simulink model "PubIfDecisionTOS_MDL"  (R2020b)
settings: configuration reference "DspaceConfig" (kept outside this file)
PostLoadFcn:
  | if any(exist('dsrtsu_mdlpostloadfcn', 'file') ~= 0), dsrtsu_mdlpostloadfcn('Execute', bdroot); end
InitFcn:
  | , if any(exist('dsmpb_private', 'file') ~= 0), dsmpb_private('dsmpb_mdlclblib', 'Init', bdroot); end,
undefined symbols (not defined in the file or in its folder): C_TOS_ACCEgoRAxletoFbumplength_m, C_TOS_ACCTargetFront_Flag, C_TOS_AEBJAPedObjDxThre_Val, C_TOS_AEBJAPedObjDyThre_Val, C_TOS_AEBJATargetSize_Val, C_TOS_AEBJAVehObjDxThre_Val, C_TOS_AEBJAVehObjDyThre_Val, C_TOS_AEBJuncPedTargetSize_Val, C_TOS_AEBLatObjDxThre_Val, C_TOS_AEBLatPedDyThre_Val, C_TOS_AEBLatTargetSize_Val, C_TOS_AEBLongTargetInEgoFront_Flag, C_TOS_axAbsGround_Parameter, C_TOS_CameraConfirmedFlag, C_TOS_CNsubjWidth, C_TOS_CurrentLaneCoreMinWidth_Val, C_TOS_CutInProb_Val_Zero, C_TOS_CutOutProb_Val_Zero, C_TOS_D2R_Val, C_TOS_DefaultValueObjectToCenterLine_dy, C_TOS_EgoCarWidth_Val, C_TOS_EgoDxRefPoint_m, C_TOS_EgoRAxletoFbumplength_m, C_TOS_HalfWidthVehicle_Con, C_TOS_HWA_CurrentLaneFlag, C_TOS_HWA_LeftLaneFlag, C_TOS_HWA_MovingDir_Vaild, C_TOS_HWA_MovState_Vaild, C_TOS_HWA_RightLaneFlag, C_TOS_LaneLineCourseErrorFront, C_TOS_LaneLineCourseErrorRear, C_TOS_MotorbikeDefaultWidth_m, C_TOS_NumberOfEffectiveTargets, C_TOS_Obj_Age_Val, C_TOS_Objdx_Constraint_Val, C_TOS_ObjectDefaultWidth_m, C_TOS_ObjInCurrentLane_Val, C_TOS_ObjInCurrentLaneValid, C_TOS_ObjInLeftLaneValid, C_TOS_ObjInRightLaneValid, C_TOS_ObjNotInCurrentLane_Val, C_TOS_ObjNotREElementType, C_TOS_ObjPredictDis_dy_ConstantVal_Zeros, C_TOS_ObjToCenterLine_ConstantVal_Zeros, C_TOS_OFMObjIDInvilad_Val, C_TOS_PIL_LatDisCons_Val_zero, C_TOS_PIL_ObjectCutInFlag_b, C_TOS_PIL_ObjectCutOutFlag_b, C_TOS_PIL_ObjLaneProb_al_Val, C_TOS_PP_ObjFusType_FC_Confirm_b, C_TOS_PP_ObjFusType_FC_FR_Confirm_b, C_TOS_PP_ObjFusType_FR_Confirm_b, C_TOS_RE_80BoolDefault_Val, C_TOS_RE_80Single181Default_Val, C_TOS_RE_80Single255Default_Val, C_TOS_RE_80Uint8Default_Val, C_TOS_RE_D2R, C_TOS_RE_D_180_Val, C_TOS_RE_InvalidObjectID_Val, C_TOS_RE_InvalidTargetChainDir_Val ... (+142)
libraries: simulink x1650, TOS_LIB x361, canfdmsglib x14
(part 67 of 69)

== stateflow chart PubIfDecisionTOS_MDL/TOS_20201112/TOS_2012080320/PP1128/AAT-AdditionalAttributes/RoadEdge/RE_2020_12_07/RoadEdge_V2/TargetChain/ObjectIsTargetChainElement/EgoLeft_TargetChainElementJudge ==
  state TargetChainElementJudge [function]
    (default) -> (junction 511) : {
        | OFM_Target_Index_i = RE_StationaryObjectsSortIndex[i] - uint8(1);
        | OFM_Target_Index_i_1  = RE_StationaryObjectsSortIndex[i- uint8(1)] - uint8(1);
        |  }
        | %OFM目标的 Index,从0开始
    (junction 511) -> (junction 327)
    (junction 327) -> (junction 333) [order 1] : [(i == uint8(1)&&RE_TargetChainStartDirection[i] == uint8(1))||...
        | RE_TargetChainDirection[i] == uint8(1)||...
        | RE_TargetChainDirection[i] == uint8(3)||...
        | RE_TargetChainDirection[i] == uint8(5)]
    (junction 327) -> (junction 357) [order 2]
    (junction 333) -> (junction 337)
    (junction 337) -> (junction 332) [order 1] : [abs(Object_Dx[OFM_Target_Index_i] - Object_Dx[OFM_Target_Index_i_1]) < P_TOS_RE_SameDirTargetChainDxThre_Val&&...
        | abs(Object_Dy[OFM_Target_Index_i] - Object_Dy[OFM_Target_Index_i_1]) <P_TOS_RE_SameDirTargetChainDyThre_Val]
    (junction 357) -> (junction 352) [order 1] : [(i == uint8(1)&&(RE_TargetChainStartDirection[i] == uint8(2)||...
        | RE_TargetChainStartDirection[i] == uint8(3)))||...
        | RE_TargetChainDirection[i] == uint8(2)||...
        | RE_TargetChainDirection[i] == uint8(4)||...
        | RE_TargetChainDirection[i] == uint8(6)]
    (junction 332) -> (junction 353) : {
        | RE_TargetChainElementFlag[i] = true;
        | }
    (junction 352) -> (junction 349)
    (junction 337) -> (junction 331) [order 2] : {
        | RE_TargetChainElementFlag[i] = false;
        | }
    (junction 357) -> (junction 336) [order 2] : {
        | RE_TargetChainElementFlag[i] = false;
        | }
    (junction 349) -> (junction 356) [order 1] : [abs(Object_Dx[OFM_Target_Index_i] - Object_Dx[OFM_Target_Index_i_1] )< P_TOS_RE_DiffDirTargetChainDxThre_Val&&...
        | abs(Object_Dy[OFM_Target_Index_i] - Object_Dy[OFM_Target_Index_i_1] )<P_TOS_RE_DiffDirTargetChainDyThre_Val]
    (junction 349) -> (junction 355) [order 2] : {
        | RE_TargetChainElementFlag[i] = false;
        | }
    (junction 356) -> (junction 329) : {
        | RE_TargetChainElementFlag[i] = true;
        | }
    (junction 355) -> (junction 336)
    (junction 329) -> (junction 355)
    (junction 331) -> (junction 329)
    (junction 353) -> (junction 331)
    (junction 336) -> (junction 460)
  state TargetChainNumCal [function]
    note: 计算连续满足条件的元素个数
    note: 3个目标组成一条链目标连；
        | 计算得到目标链的起始目标在Dx排序中的Index+1；
    (default) -> (junction 372)
    (junction 372) -> (junction 378) [order 1] : [RE_TargetChainElementFlag[i] == true]
    (junction 372) -> (junction 379) [order 2] : {
        | ElementCounter[i] = uint8(0);
        | }
    (junction 378) -> (junction 396) : {
        | ElementCounter[i] = ElementCounter[i-uint8(1)] + uint8(1);
        | }
    (junction 396) -> (junction 379)
    (junction 379) -> (junction 369)
    (junction 369) -> (junction 382) [order 1] : [ElementCounter[i] == uint8(2)]
        | %连续2个目标符合条件时，从起始目标到当前目标一共是3个目标；
    (junction 369) -> (junction 375) [order 2]
    (junction 382) -> (junction 376) : {
        | TargetChainStartIndex[i - uint8(2)] = i - uint8(1);
        | TargetChainStartIndex[i - uint8(1)] = i - uint8(1);
        | TargetChainStartIndex[i] = i - uint8(1);
        | %ElementCounter[i - uint8(2)] == uint8(1);
        | %ElementCounter[i - uint8(1)] == uint8(2);
        | %目标链开始元素从1开始计数
        | }
    (junction 375) -> (junction 373) [order 1] : [ElementCounter[i] > uint8(2)]
    (junction 375) -> (junction 377) [order 2] : {
        | TargetChainStartIndex[i] = uint8(0);
        | %ElementCounter[i] = uint8(0);
        | }
    (junction 373) -> (junction 387) : {
        | TargetChainStartIndex[i] = TargetChainStartIndex[i - uint8(1)];
        | }
    (junction 387) -> (junction 377)
    (junction 376) -> (junction 387)
    (junction 377) -> (junction 495)
  (default) -> (junction 2) : {
      | i = uint8(1);
      | RE_TargetChainElementFlag = C_TOS_RE_80BoolDefault_Val;
      | TargetChainStartIndex = C_TOS_RE_80Uint8Default_Val;
      | ElementCounter = C_TOS_RE_80Uint8Default_Val;
      | }
      | %从第2个目标开始
  (junction 2) -> (junction 3) [order 1] : [RE_StationaryObjectsSortIndex[i] ~= C_TOS_StillObjSortInvalidIndex_Val&&...
      | i <= uint8(79)]
  (junction 360) -> (junction 2) : {
      | i = i+uint8(1);
      | }
  (junction 2) -> (junction 314) [order 2]
  (junction 3) -> (junction 358) : {
      | TargetChainElementJudge();
      | }
  (junction 358) -> (junction 360) : {
      | TargetChainNumCal();
      | }
  (junction 314) -> (junction 8)
  data: C_TOS_RE_InvalidTargetChainDir_Val parameter; C_TOS_StillObjSortInvalidIndex_Val parameter; Object_Dx input; Object_Dy input; P_TOS_RE_DiffDirTargetChainDxThre_Val parameter; P_TOS_RE_DiffDirTargetChainDyThre_Val parameter; P_TOS_RE_SameDirTargetChainDxThre_Val parameter; P_TOS_RE_SameDirTargetChainDyThre_Val parameter; RE_StationaryObjectsSortIndex input; RE_TargetChainDirection input; RE_TargetChainStartDirection input; i local uint8 =; RE_TargetChainElementFlag output boolean size=80; TargetChainStartIndex output uint8 size=80; OFM_Target_Index_i local uint8 size=1; k local uint8; TargetChainNum local uint8; OFM_Target_Index_i_1 local uint8 size=1; C_TOS_RE_80BoolDefault_Val parameter; C_TOS_RE_80Uint8Default_Val parameter; ElementCounter output uint8 size=80 =

== stateflow chart PubIfDecisionTOS_MDL/TOS_20201112/TOS_2012080320/PP1128/AAT-AdditionalAttributes/RoadEdge/RE_2020_12_07/RoadEdge_V2/TargetChain/ObjectIsTargetChainElement/EgoLeft_TargetChainInfor ==
  state TargetChainNumCal [function]
    note: 给目标链编号
    (default) -> (junction 473) : %目标链条数从1开始
    (junction 473) -> (junction 482) [order 1] : [i == uint8(0)]
    (junction 473) -> (junction 374) [order 2]
    (junction 482) -> (junction 481)
    (junction 374) -> (junction 383) [order 1] : [(TargetChainStartIndex[i-uint8(1)] == uint8(0)&&...
        | TargetChainStartIndex[i] != uint8(0))||...
        | (TargetChainStartIndex[i-uint8(1)] != uint8(0)&&...
        | TargetChainStartIndex[i] != uint8(0)&&...
        | TargetChainStartIndex[i] != TargetChainStartIndex[i-uint8(1)])]
        | %目标链开始元素
    (junction 481) -> (junction 475) [order 1] : [TargetChainStartIndex[i] != uint8(0)]
        | %Dx最近的目标是目标链开始元素
    (junction 374) -> (junction 365) [order 2]
    (junction 383) -> (junction 391) : {
        | TargetChainIndex[i] = TargetChainNum;
        |  TargetChainNum = TargetChainNum + uint8(1);
        | }
    (junction 481) -> (junction 486) [order 2] : {
        | TargetChainIndex[i] = uint8(0);
        | }
    (junction 475) -> (junction 477) : {
        | TargetChainIndex[i] = TargetChainNum;
        |  TargetChainNum = TargetChainNum + uint8(1);
        | }
    (junction 365) -> (junction 414) [order 1] : [TargetChainStartIndex[i] != uint8(0)&&...
        | TargetChainStartIndex[i] == TargetChainStartIndex[i-uint8(1)]]
        | %目标链剩余元素
    (junction 365) -> (junction 381) [order 2] : {
        | TargetChainIndex[i] = uint8(0);
        | }
    (junction 414) -> (junction 368) : {
        | TargetChainIndex[i] = TargetChainIndex[i-uint8(1)];
        | }
    (junction 368) -> (junction 381)
    (junction 391) -> (junction 368)
    (junction 486) -> (junction 391)
    (junction 477) -> (junction 486)
    (junction 381) -> (junction 501)
  state TargetChainElementNumCal [function]
    (default) -> (junction 517)
    (junction 517) -> (junction 516) [order 1] : [i > uint8(0)]
    (junction 517) -> (junction 520) [order 2] : {
        | TargetChainElementNum[i] = uint8(0);
        | }
    (junction 516) -> (junction 437)
    (junction 437) -> (junction 448) [order 1] : [(TargetChainStartIndex[i-uint8(1)] != uint8(0)&&...
        | TargetChainStartIndex[i] == uint8(0))||...
        | (TargetChainStartIndex[i-uint8(1)] != uint8(0)&&...
        | TargetChainStartIndex[i] != TargetChainStartIndex[i-uint8(1)])]
        | %[i-uint8(1)]为目标链结束元素
    (junction 437) -> (junction 442) [order 2] : {
        | TargetChainElementNum[i-uint8(1)] = uint8(0);
        | }
    (junction 448) -> (junction 453) : {
        | TargetChainElementNum[i-uint8(1)] = ElementCounter[i-uint8(1)] + uint8(1);
        | }
    (junction 442) -> (junction 520)
    (junction 453) -> (junction 442)
    (junction 520) -> (junction 524)
    (junction 524) -> (junction 525) [order 1] : [i > uint8(2)&&TargetChainElementNum[i-uint8(1)]  != uint8(0)]
        | %目标链结束元素，从第3个目标开始判断，[i]目标为目标链结束元素
    (junction 524) -> (junction 527) [order 2] : %donothing
    (junction 525) -> (junction 534) : {
        | j = uint8(1);
        | }
    (junction 534) -> (junction 536) [order 1] : [ j<=TargetChainElementNum[i-uint8(1)] ]
    (junction 538) -> (junction 534) : {
        | j = j+uint8(1);
        | }
    (junction 534) -> (junction 529) [order 2]
    (junction 536) -> (junction 538) : {
        | TargetChainElementNum[i-j] = TargetChainElementNum[i-uint8(1)];
        | }
        | %同一目标链上所有元素标记目标链的元素个数
    (junction 529) -> (junction 527)
    (junction 527) -> (junction 532)
  (default) -> (junction 2) : {
      | i = uint8(0);
      | TargetChainIndex = C_TOS_RE_80Uint8Default_Val;
      | TargetChainElementNum = C_TOS_RE_80Uint8Default_Val;
      | TargetChainNum=uint8(1);
      | }
      | %从第1个目标开始
  (junction 2) -> (junction 3) [order 1] : [(RE_StationaryObjectsSortIndex[i] ~= C_TOS_StillObjSortInvalidIndex_Val||...
      | (i > uint8(0)&&RE_StationaryObjectsSortIndex[i-uint8(1)] ~= C_TOS_StillObjSortInvalidIndex_Val))&&...
      | i <= uint8(79)]
      | %循环到有效目标的下一个目标，保证找到目标链的结束元素
  (junction 273) -> (junction 2) : {
      | i = i+uint8(1);
      | }
  (junction 2) -> (junction 314) [order 2]
  (junction 3) -> (junction 360) : {
      | TargetChainNumCal();
      | }
  (junction 360) -> (junction 273) : {
      | TargetChainElementNumCal();
      | }
  (junction 314) -> (junction 8)
  data: RE_StationaryObjectsSortIndex input; TargetChainStartIndex input; i local uint8 size=1 =; TargetChainIndex output uint8 size=80; TargetChainElementNum output uint8 size=80; TargetChainNum local uint8 size=1 =1; C_TOS_RE_80BoolDefault_Val parameter; C_TOS_RE_80Uint8Default_Val parameter; ElementCounter input uint8 size=80 =; C_TOS_StillObjSortInvalidIndex_Val parameter; j local uint8 size=1

== stateflow chart PubIfDecisionTOS_MDL/TOS_20201112/TOS_2012080320/PP1128/AAT-AdditionalAttributes/RoadEdge/RE_2020_12_07/RoadEdge_V2/TargetChain/ObjectIsTargetChainElement/EgoRight_TargetChainElementJudge ==
  state TargetChainElementJudge [function]
    (default) -> (junction 511) : {
        | OFM_Target_Index_i = RE_StationaryObjectsSortIndex[i] - uint8(1);
        | OFM_Target_Index_i_1  = RE_StationaryObjectsSortIndex[i- uint8(1)] - uint8(1);
        |  }
        | %OFM目标的 Index,从0开始
    (junction 511) -> (junction 327)
    (junction 327) -> (junction 333) [order 1] : [(i == uint8(1)&&RE_TargetChainStartDirection[i] == uint8(1))||...
        | RE_TargetChainDirection[i] == uint8(1)||...
        | RE_TargetChainDirection[i] == uint8(3)||...
        | RE_TargetChainDirection[i] == uint8(5)]
    (junction 327) -> (junction 357) [order 2]
    (junction 333) -> (junction 337)
    (junction 337) -> (junction 332) [order 1] : [abs(Object_Dx[OFM_Target_Index_i] - Object_Dx[OFM_Target_Index_i_1]) < P_TOS_RE_SameDirTargetChainDxThre_Val&&...
        | abs(Object_Dy[OFM_Target_Index_i] - Object_Dy[OFM_Target_Index_i_1]) <P_TOS_RE_SameDirTargetChainDyThre_Val]
    (junction 357) -> (junction 352) [order 1] : [(i == uint8(1)&&(RE_TargetChainStartDirection[i] == uint8(2)||...
        | RE_TargetChainStartDirection[i] == uint8(3)))||...
        | RE_TargetChainDirection[i] == uint8(2)||...
        | RE_TargetChainDirection[i] == uint8(4)||...
        | RE_TargetChainDirection[i] == uint8(6)]
    (junction 332) -> (junction 353) : {
        | RE_TargetChainElementFlag[i] = true;
        | }
    (junction 352) -> (junction 349)
    (junction 337) -> (junction 331) [order 2] : {
        | RE_TargetChainElementFlag[i] = false;
        | }
    (junction 357) -> (junction 336) [order 2] : {
        | RE_TargetChainElementFlag[i] = false;
        | }
    (junction 349) -> (junction 356) [order 1] : [abs(Object_Dx[OFM_Target_Index_i] - Object_Dx[OFM_Target_Index_i_1] )< P_TOS_RE_DiffDirTargetChainDxThre_Val&&...
        | abs(Object_Dy[OFM_Target_Index_i] - Object_Dy[OFM_Target_Index_i_1] )<P_TOS_RE_DiffDirTargetChainDyThre_Val]
    (junction 349) -> (junction 355) [order 2] : {
        | RE_TargetChainElementFlag[i] = false;
        | }
    (junction 356) -> (junction 329) : {
        | RE_TargetChainElementFlag[i] = true;
        | }
    (junction 355) -> (junction 336)
    (junction 329) -> (junction 355)
    (junction 331) -> (junction 329)
    (junction 353) -> (junction 331)
    (junction 336) -> (junction 460)
  state TargetChainNumCal [function]
    note: 计算连续满足条件的元素个数
    note: 3个目标组成一条链目标连；
        | 计算得到目标链的起始目标在Dx排序中的Index+1；
    (default) -> (junction 372)
    (junction 372) -> (junction 378) [order 1] : [RE_TargetChainElementFlag[i] == true]
    (junction 372) -> (junction 379) [order 2] : {
        | ElementCounter[i] = uint8(0);
        | }
    (junction 378) -> (junction 396) : {
        | ElementCounter[i] = ElementCounter[i-uint8(1)] + uint8(1);
        | }
    (junction 396) -> (junction 379)
    (junction 379) -> (junction 369)
    (junction 369) -> (junction 382) [order 1] : [ElementCounter[i] == uint8(2)]
        | %连续2个目标符合条件时，从起始目标到当前目标一共是3个目标；
    (junction 369) -> (junction 375) [order 2]
    (junction 382) -> (junction 376) : {
        | TargetChainStartIndex[i - uint8(2)] = i - uint8(1);
        | TargetChainStartIndex[i - uint8(1)] = i - uint8(1);
        | TargetChainStartIndex[i] = i - uint8(1);
        | %ElementCounter[i - uint8(2)] == uint8(1);
        | %ElementCounter[i - uint8(1)] == uint8(2);
        | %目标链开始元素从1开始计数
        | }
    (junction 375) -> (junction 373) [order 1] : [ElementCounter[i] > uint8(2)]
    (junction 375) -> (junction 377) [order 2] : {
        | TargetChainStartIndex[i] = uint8(0);
        | %ElementCounter[i] = uint8(0);
        | }
    (junction 373) -> (junction 387) : {
        | TargetChainStartIndex[i] = TargetChainStartIndex[i - uint8(1)];
        | }
    (junction 387) -> (junction 377)
    (junction 376) -> (junction 387)
    (junction 377) -> (junction 495)
  (default) -> (junction 2) : {
      | i = uint8(1);
      | RE_TargetChainElementFlag = C_TOS_RE_80BoolDefault_Val;
      | TargetChainStartIndex = C_TOS_RE_80Uint8Default_Val;
      | ElementCounter = C_TOS_RE_80Uint8Default_Val;
      | }
      | %从第2个目标开始
  (junction 2) -> (junction 3) [order 1] : [RE_StationaryObjectsSortIndex[i] ~= C_TOS_StillObjSortInvalidIndex_Val&&...
      | i <= uint8(79)]
  (junction 360) -> (junction 2) : {
      | i = i+uint8(1);
      | }
  (junction 2) -> (junction 314) [order 2]
  (junction 3) -> (junction 358) : {
      | TargetChainElementJudge();
      | }
  (junction 358) -> (junction 360) : {
      | TargetChainNumCal();
      | }
  (junction 314) -> (junction 8)
  data: C_TOS_RE_InvalidTargetChainDir_Val parameter; C_TOS_StillObjSortInvalidIndex_Val parameter; Object_Dx input; Object_Dy input; P_TOS_RE_DiffDirTargetChainDxThre_Val parameter; P_TOS_RE_DiffDirTargetChainDyThre_Val parameter; P_TOS_RE_SameDirTargetChainDxThre_Val parameter; P_TOS_RE_SameDirTargetChainDyThre_Val parameter; RE_StationaryObjectsSortIndex input; RE_TargetChainDirection input; RE_TargetChainStartDirection input; i local uint8 =; RE_TargetChainElementFlag output boolean size=80; TargetChainStartIndex output uint8 size=80; OFM_Target_Index_i local uint8 size=1; k local uint8; TargetChainNum local uint8; OFM_Target_Index_i_1 local uint8 size=1; C_TOS_RE_80BoolDefault_Val parameter; C_TOS_RE_80Uint8Default_Val parameter; ElementCounter output uint8 size=80 =

== stateflow chart PubIfDecisionTOS_MDL/TOS_20201112/TOS_2012080320/PP1128/AAT-AdditionalAttributes/RoadEdge/RE_2020_12_07/RoadEdge_V2/TargetChain/ObjectIsTargetChainElement/EgoRight_TargetChainInfor ==
  state TargetChainNumCal [function]
    note: 给目标链编号
    (default) -> (junction 473) : %目标链条数从1开始
    (junction 473) -> (junction 482) [order 1] : [i == uint8(0)]
    (junction 473) -> (junction 374) [order 2]
    (junction 482) -> (junction 481)
    (junction 374) -> (junction 383) [order 1] : [(TargetChainStartIndex[i-uint8(1)] == uint8(0)&&...
        | TargetChainStartIndex[i] != uint8(0))||...
        | (TargetChainStartIndex[i-uint8(1)] != uint8(0)&&...
        | TargetChainStartIndex[i] != uint8(0)&&...
        | TargetChainStartIndex[i] != TargetChainStartIndex[i-uint8(1)])]
        | %目标链开始元素
    (junction 481) -> (junction 475) [order 1] : [TargetChainStartIndex[i] != uint8(0)]
        | %Dx最近的目标是目标链开始元素
    (junction 374) -> (junction 365) [order 2]
    (junction 383) -> (junction 391) : {
        | TargetChainIndex[i] = TargetChainNum;
        |  TargetChainNum = TargetChainNum + uint8(1);
        | }
    (junction 481) -> (junction 486) [order 2] : {
        | TargetChainIndex[i] = uint8(0);
        | }
    (junction 475) -> (junction 477) : {
        | TargetChainIndex[i] = TargetChainNum;
        |  TargetChainNum = TargetChainNum + uint8(1);
        | }
    (junction 365) -> (junction 414) [order 1] : [TargetChainStartIndex[i] != uint8(0)&&...
        | TargetChainStartIndex[i] == TargetChainStartIndex[i-uint8(1)]]
        | %目标链剩余元素
    (junction 365) -> (junction 381) [order 2] : {
        | TargetChainIndex[i] = uint8(0);
        | }
    (junction 414) -> (junction 368) : {
        | TargetChainIndex[i] = TargetChainIndex[i-uint8(1)];
        | }
    (junction 368) -> (junction 381)
    (junction 391) -> (junction 368)
    (junction 486) -> (junction 391)
    (junction 477) -> (junction 486)
    (junction 381) -> (junction 501)
  state TargetChainElementNumCal [function]
    (default) -> (junction 517)
    (junction 517) -> (junction 516) [order 1] : [i > uint8(0)]
    (junction 517) -> (junction 520) [order 2] : {
        | TargetChainElementNum[i] = uint8(0);
        | }
    (junction 516) -> (junction 437)
    (junction 437) -> (junction 448) [order 1] : [(TargetChainStartIndex[i-uint8(1)] != uint8(0)&&...
        | TargetChainStartIndex[i] == uint8(0))||...
        | (TargetChainStartIndex[i-uint8(1)] != uint8(0)&&...
        | TargetChainStartIndex[i] != TargetChainStartIndex[i-uint8(1)])]
        | %[i-uint8(1)]为目标链结束元素
    (junction 437) -> (junction 442) [order 2] : {
        | TargetChainElementNum[i-uint8(1)] = uint8(0);
        | }
    (junction 448) -> (junction 453) : {
        | TargetChainElementNum[i-uint8(1)] = ElementCounter[i-uint8(1)] + uint8(1);
        | }
    (junction 442) -> (junction 520)
    (junction 453) -> (junction 442)
    (junction 520) -> (junction 524)
    (junction 524) -> (junction 525) [order 1] : [i > uint8(2)&&TargetChainElementNum[i-uint8(1)]  != uint8(0)]
        | %目标链结束元素，从第3个目标开始判断，[i]目标为目标链结束元素
    (junction 524) -> (junction 527) [order 2] : %donothing
    (junction 525) -> (junction 534) : {
        | j = uint8(1);
        | }
    (junction 534) -> (junction 536) [order 1] : [ j<=TargetChainElementNum[i-uint8(1)] ]
    (junction 538) -> (junction 534) : {
        | j = j+uint8(1);
        | }
    (junction 534) -> (junction 529) [order 2]
    (junction 536) -> (junction 538) : {
        | TargetChainElementNum[i-j] = TargetChainElementNum[i-uint8(1)];
        | }
        | %同一目标链上所有元素标记目标链的元素个数
    (junction 529) -> (junction 527)
    (junction 527) -> (junction 532)
  (default) -> (junction 2) : {
      | i = uint8(0);
      | TargetChainIndex = C_TOS_RE_80Uint8Default_Val;
      | TargetChainElementNum = C_TOS_RE_80Uint8Default_Val;
      | TargetChainNum=uint8(1);
      | }
      | %从第1个目标开始
  (junction 2) -> (junction 3) [order 1] : [(RE_StationaryObjectsSortIndex[i] ~= C_TOS_StillObjSortInvalidIndex_Val||...
      | (i > uint8(0)&&RE_StationaryObjectsSortIndex[i-uint8(1)] ~= C_TOS_StillObjSortInvalidIndex_Val))&&...
      | i <= uint8(79)]
      | %循环到有效目标的下一个目标，保证找到目标链的结束元素
  (junction 273) -> (junction 2) : {
      | i = i+uint8(1);
      | }
  (junction 2) -> (junction 314) [order 2]
  (junction 3) -> (junction 360) : {
      | TargetChainNumCal();
      | }
  (junction 360) -> (junction 273) : {
      | TargetChainElementNumCal();
      | }
  (junction 314) -> (junction 8)
  data: RE_StationaryObjectsSortIndex input; TargetChainStartIndex input; i local uint8 size=1 =; TargetChainIndex output uint8 size=80; TargetChainElementNum output uint8 size=80; TargetChainNum local uint8 size=1 =1; C_TOS_RE_80BoolDefault_Val parameter; C_TOS_RE_80Uint8Default_Val parameter; ElementCounter input uint8 size=80 =; C_TOS_StillObjSortInvalidIndex_Val parameter; j local uint8 size=1

== stateflow chart PubIfDecisionTOS_MDL/TOS_20201112/TOS_2012080320/TOS/AEB/TOS_AEBJunct_20201208/AEBJunctionTargetInfor/AEBJuncTargetObjectType/AEBJuncTargetObjectType/TOS_AEBJunc_TargetObjectType ==
  state AEBJuncSameTargetType [function]
    (default) -> (junction 39) : {
        | i = uint8(1);
        | AEBJunc_TargetObjectType = OFM_OBJ_TYPE_E.INVALID;
        | }
    (junction 39) -> (junction 40) [order 1] : [i<=C_TOS_AEBJATargetSize_Val]
    (junction 45) -> (junction 39)
    (junction 39) -> (junction 46) [order 2]
    (junction 40) -> (junction 41)
    (junction 41) -> (junction 42) [order 1] : [AEBJunc_Target_ObjectID_K1(i) == Object_ID]
    (junction 41) -> (junction 43) [order 2] : %donothing
    (junction 42) -> (junction 44) : {
        | AEBJunc_TargetObjectType = AEBJunc_Target_ObjectType_K1(i);
        | i = C_TOS_AEBJATargetSize_Val+uint8(1);
        | }
    (junction 44) -> (junction 43)
    (junction 43) -> (junction 45) : {i = i+uint8(1);}
  (default) -> (junction 1)
  (junction 1) -> (junction 5) [order 1] : [ObjectType == OFM_OBJ_TYPE_E.PEDESTRIAN||...
      | ObjectType == OFM_OBJ_TYPE_E.BICYCLE||...
      | ObjectType == OFM_OBJ_TYPE_E.MOTORBIKE||...
      | ObjectType == OFM_OBJ_TYPE_E.CAR||...
      | ObjectType == OFM_OBJ_TYPE_E.TRUCK]
  (junction 1) -> (junction 27) [order 2] : {
      | AEBJuncSameTargetType();
      | }
  (junction 5) -> (junction 26) : {
      | AEBJunc_TargetObjectType = ObjectType;
      | }
  (junction 26) -> (junction 27)
  (junction 27) -> (junction 30)
  data: ObjectType input Enum: OFM_OBJ_TYPE_E size=1; Object_ID input uint8 size=1; AEBJunc_Target_ObjectType_K1 input Enum: OFM_OBJ_TYPE_E size=32; AEBJunc_Target_ObjectID_K1 input uint8 size=32; AEBJunc_TargetObjectType output Enum: OFM_OBJ_TYPE_E size=1; C_TOS_AEBJATargetSize_Val parameter

== stateflow chart PubIfDecisionTOS_MDL/TOS_20201112/TOS_2012080320/TOS/AEB/TOS_AEBJunct_20201208/AEBJunctionTargetInfor/TOS_AEBJunct ==
  (default) -> (junction 1) : {i=uint8(1);}
  (junction 1) -> (junction 40) [order 1] : [i<=C_TOS_AEBJATargetSize_Val]
  (junction 42) -> (junction 1) : {i=i+uint8(1);}
  (junction 1) -> (junction 60) [order 2]
  (junction 40) -> (junction 42) : {
      | TOS_AEBJuncTargetBus(i).FusionType= uint8(0);
      | TOS_AEBJuncTargetBus(i).ObjectID= uint8(0);
      | TOS_AEBJuncTargetBus(i).ObjectType= uint8(0);
      | TOS_AEBJuncTargetBus(i).ObjectTypeCameraConfirmed= false;
      | TOS_AEBJuncTargetBus(i).ObjectLength=single(0);
      | TOS_AEBJuncTargetBus(i).ObjectWidth= single(0);
      | TOS_AEBJuncTargetBus(i).ObjectHight= single(0);
      | TOS_AEBJuncTargetBus(i).ObjectYawAngle= single(0);
      | TOS_AEBJuncTargetBus(i).ObjectAzimuthAngle= single(0);
      | TOS_AEBJuncTargetBus(i).ObjectMovingState= uint8(0);
      | TOS_AEBJuncTargetBus(i).ObjectMovingOrientation=uint8(0);
      | TOS_AEBJuncTargetBus(i).dxFisrtDetection= single(0);
      | TOS_AEBJuncTargetBus(i).dyFisrtDetection= single(0);
      | TOS_AEBJuncTargetBus(i).dx= single(0);
      | TOS_AEBJuncTargetBus(i).dy= single(0);
      | TOS_AEBJuncTargetBus(i).dz= single(0);
      | TOS_AEBJuncTargetBus(i).vx= single(0);
      | TOS_AEBJuncTargetBus(i).vy= single(0);
      | TOS_AEBJuncTargetBus(i).ax= single(0);
      | TOS_AEBJuncTargetBus(i).ay= single(0);
      | TOS_AEBJuncTargetBus(i).dxVariance= single(0);
      | TOS_AEBJuncTargetBus(i).dyVariance= single(0);
      | TOS_AEBJuncTargetBus(i).vxVariance= single(0);
      | TOS_AEBJuncTargetBus(i).vyVariance= single(0);
      | TOS_AEBJuncTargetBus(i).axVariance= single(0);
      | TOS_AEBJuncTargetBus(i).ayVariance= single(0);
      | TOS_AEBJuncTargetBus(i).ObjectLengthVar= single(0);
      | TOS_AEBJuncTargetBus(i).ObjectWidthVar= single(0);
      | TOS_AEBJuncTargetBus(i).ObjectYawAngleVar= single(0);
      | TOS_AEBJuncTargetBus(i).ObjectTypeProb= single(0);
      | TOS_AEBJuncTargetBus(i).ObjectMovingStateProb= single(0);
      | TOS_AEBJuncTargetBus(i).ObjectMovingOrientationProb= single(0);
      | TOS_AEBJuncTargetBus(i).ObjectExistProb= single(0);
      | TOS_AEBJuncTargetBus(i).ObjectIsObstacleProb= single(0);
      | TOS_AEBJuncTargetBus(i).ObjectRCS= single(0);
      | TOS_AEBJuncTargetBus(i).ObjectMeasurementStatus= single(0);
      | TOS_AEBJuncTargetBus(i).ObjectLifeCycle= uint16(0);
      | TOS_AEBJuncTargetBus(i).ObjUpdate= false;
      | }
  (junction 60) -> (junction 53) : {i=uint8(1);
      | j=uint8(1);}
  (junction 53) -> (junction 62) [order 1] : [i<=C_TOS_AEBJATargetSize_Val]
  (junction 66) -> (junction 53) : {i=i+uint8(1);}
  (junction 53) -> (junction 46) [order 2]
  (junction 62) -> (junction 64)
  (junction 64) -> (junction 3) [order 1] : [TOS_AEBJATargetIndex(i)~=uint8(0)]
  (junction 64) -> (junction 66) [order 2]
  (junction 3) -> (junction 5) : {
      | TargetIndex = TOS_AEBJATargetIndex(i);
      | TOS_AEBJuncTargetBus(j).FusionType=OFM_SignalVerification.Object_Fus_Type(TargetIndex);
      | TOS_AEBJuncTargetBus(j).ObjectID=OFM_SignalVerification.Object_ID(TargetIndex);
      | TOS_AEBJuncTargetBus(j).ObjectType=AEBJuncTargetObjectType(i);
      | TOS_AEBJuncTargetBus(j).ObjectTypeCameraConfirmed=TOS_AddAttributes.PP_CamareConfirmSignalProcessing(TargetIndex);
      | TOS_AEBJuncTargetBus(j).ObjectLength=OFM_SignalVerification.Object_Length(TargetIndex);
      | TOS_AEBJuncTargetBus(j).ObjectWidth=OFM_SignalVerification.Object_Width(TargetIndex);
      | TOS_AEBJuncTargetBus(j).ObjectHight=OFM_SignalVerification.Object_Hight(TargetIndex);
      | TOS_AEBJuncTargetBus(j).ObjectYawAngle=OFM_SignalVerification.Object_HeadingAngle(TargetIndex);
      | TOS_AEBJuncTargetBus(j).ObjectAzimuthAngle=OFM_SignalVerification.Object_YawAngle(TargetIndex);
      | TOS_AEBJuncTargetBus(j).ObjectMovingState=TOS_AddAttributes.PP_MovingState_AEB_SignalProcessing(TargetIndex);
      | TOS_AEBJuncTargetBus(j).ObjectMovingOrientation=TOS_AddAttributes.PP_ObjMovingDirSignalProcessing(TargetIndex);
      | TOS_AEBJuncTargetBus(j).dxFisrtDetection=TOS_AddAttributes.PP_ObjFirstDetect_Dx(TargetIndex);
      | TOS_AEBJuncTargetBus(j).dyFisrtDetection=TOS_AddAttributes.PP_ObjFirstDetect_Dy(TargetIndex);
      | TOS_AEBJuncTargetBus(j).dx=OFM_SignalVerification.Object_DX(TargetIndex);
      | TOS_AEBJuncTargetBus(j).dy=OFM_SignalVerification.Object_DY(TargetIndex);
      | TOS_AEBJuncTargetBus(j).dz= single(0);
      | TOS_AEBJuncTargetBus(j).vx=OFM_SignalVerification.Object_VX(TargetIndex);
      | TOS_AEBJuncTargetBus(j).vy=OFM_SignalVerification.Object_VY(TargetIndex);
      | TOS_AEBJuncTargetBus(j).ax=OFM_SignalVerification.Object_AX(TargetIndex);
      | TOS_AEBJuncTargetBus(j).ay=OFM_SignalVerification.Object_AY(TargetIndex);
      | TOS_AEBJuncTargetBus(j).dxVariance=OFM_SignalVerification.Object_Std_DX(TargetIndex);
      | TOS_AEBJuncTargetBus(j).dyVariance=OFM_SignalVerification.Object_Std_DY(TargetIndex);
      | TOS_AEBJuncTargetBus(j).vxVariance=OFM_SignalVerification.Object_Std_VX(TargetIndex);
      | TOS_AEBJuncTargetBus(j).vyVariance=OFM_SignalVerification.Object_Std_VY(TargetIndex);
      | TOS_AEBJuncTargetBus(j).axVariance=OFM_SignalVerification.Object_Std_AX(TargetIndex);
      | TOS_AEBJuncTargetBus(j).ayVariance=OFM_SignalVerification.Object_Std_AY(TargetIndex);
      | TOS_AEBJuncTargetBus(j).ObjectLengthVar=OFM_SignalVerification.Object_Std_Length(TargetIndex);
      | TOS_AEBJuncTargetBus(j).ObjectWidthVar=OFM_SignalVerification.Object_Std_Width(TargetIndex);
      | TOS_AEBJuncTargetBus(j).ObjectYawAngleVar=OFM_SignalVerification.Object_Std_HeadingAngle(TargetIndex);
      | TOS_AEBJuncTargetBus(j).ObjectTypeProb=OFM_SignalVerification.Object_Type_Prob(TargetIndex);
      | TOS_AEBJuncTargetBus(j).ObjectMovingStateProb= single(0);
      | TOS_AEBJuncTargetBus(j).ObjectMovingOrientationProb= single(0);
      | TOS_AEBJuncTargetBus(j).ObjectExistProb=OFM_SignalVerification.Object_ExistProb(TargetIndex);
      | TOS_AEBJuncTargetBus(j).ObjectIsObstacleProb=OFM_SignalVerification.Object_ObstacleProb(TargetIndex);
      | TOS_AEBJuncTargetBus(j).ObjectRCS= single(0);
      | TOS_AEBJuncTargetBus(j).ObjectMeasurementStatus= single(0);
      | TOS_AEBJuncTargetBus(j).ObjectLifeCycle=OFM_SignalVerification.Object_Age(TargetIndex);
      | TOS_AEBJuncTargetBus(j).ObjUpdate= false;
      | j=j+uint8(1);
      | }
  (junction 5) -> (junction 66)
  data: TOS_AddAttributes input Bus: TOS_AddAttributes_BUS; OFM_SignalVerification input Bus: OFM_OBJ_BUS; AEBJuncTargetObjectType input uint8; TOS_AEBJATargetIndex input uint8; TOS_AEBJuncTargetBus output Bus: TOS_AEB_JAOBJ_BUS size=32 =0; C_TOS_AEBJATargetSize_Val parameter; TargetIndex local uint8 size=1; i local uint8 size=1; j local uint8 size=1

== stateflow chart PubIfDecisionTOS_MDL/TOS_20201112/TOS_2012080320/TOS/AEB/TOS_AEBLatCro1105/AEBLatTrgInfor/AEBLatTargetObjectType/AEBLatTargetObjectType/TOS_AEBLat_TargetObjectType ==
  state AEBLatSameTargetType [function]
    (default) -> (junction 39) : {
        | i = uint8(1);
        | AEBLat_TargetObjectType = OFM_OBJ_TYPE_E.INVALID;
        | }
    (junction 39) -> (junction 40) [order 1] : [i<=C_TOS_AEBLatTargetSize_Val]
    (junction 45) -> (junction 39)
    (junction 39) -> (junction 46) [order 2]
    (junction 40) -> (junction 41)
    (junction 41) -> (junction 42) [order 1] : [AEBLat_Target_ObjectID_K1(i) == Object_ID]
    (junction 41) -> (junction 43) [order 2] : %donothing
    (junction 42) -> (junction 44) : {
        | AEBLat_TargetObjectType = AEBLat_Target_ObjectType_K1(i);
        | i = C_TOS_AEBLatTargetSize_Val+uint8(1);
        | }
    (junction 44) -> (junction 43)
    (junction 43) -> (junction 45) : {i = i+uint8(1);}
  (default) -> (junction 1)
  (junction 1) -> (junction 5) [order 1] : [ObjectType == OFM_OBJ_TYPE_E.PEDESTRIAN||...
      | ObjectType == OFM_OBJ_TYPE_E.BICYCLE||...
      | ObjectType == OFM_OBJ_TYPE_E.MOTORBIKE]
  (junction 1) -> (junction 27) [order 2] : {
      | AEBLatSameTargetType();
      | }
  (junction 5) -> (junction 26) : {
      | AEBLat_TargetObjectType = ObjectType;
      | }
  (junction 26) -> (junction 27)
  (junction 27) -> (junction 30)
  data: Object_ID input uint8; ObjectType input; AEBLat_Target_ObjectType_K1 input Enum: OFM_OBJ_TYPE_E; AEBLat_Target_ObjectID_K1 input uint8; AEBLat_TargetObjectType output Enum: OFM_OBJ_TYPE_E; C_TOS_AEBLatTargetSize_Val parameter

== stateflow chart PubIfDecisionTOS_MDL/TOS_20201112/TOS_2012080320/TOS/AEB/TOS_AEBLatCro1105/AEBLatTrgInfor/TOS_AEBLatCro ==
  (default) -> (junction 57) : {i=uint8(1);}
  (junction 57) -> (junction 61) [order 1] : [i<=C_TOS_AEBLatTargetSize_Val]
  (junction 64) -> (junction 57) : {i=i+uint8(1);}
  (junction 57) -> (junction 47) [order 2]
  (junction 61) -> (junction 64) : {
      | TOS_AEBLatTargetBus(i).FusionType= uint8(0);
      | TOS_AEBLatTargetBus(i).ObjectID= uint8(0);
      | TOS_AEBLatTargetBus(i).ObjectType= uint8(0);
      | TOS_AEBLatTargetBus(i).ObjectTypeCameraConfirmed= false;
      | TOS_AEBLatTargetBus(i).ObjectLength=single(0);
      | TOS_AEBLatTargetBus(i).ObjectWidth= single(0);
      | TOS_AEBLatTargetBus(i).ObjectHight= single(0);
      | TOS_AEBLatTargetBus(i).ObjectYawAngle= single(0);
      | TOS_AEBLatTargetBus(i).ObjectAzimuthAngle= single(0);
      | TOS_AEBLatTargetBus(i).ObjectMovingState= uint8(0);
      | TOS_AEBLatTargetBus(i).ObjectMovingOrientation=uint8(0);
      | TOS_AEBLatTargetBus(i).dxFisrtDetection= single(0);
      | TOS_AEBLatTargetBus(i).dyFisrtDetection= single(0);
      | TOS_AEBLatTargetBus(i).dx= single(0);
      | TOS_AEBLatTargetBus(i).dy= single(0);
      | TOS_AEBLatTargetBus(i).dz= single(0);
      | TOS_AEBLatTargetBus(i).vx= single(0);
      | TOS_AEBLatTargetBus(i).vy= single(0);
      | TOS_AEBLatTargetBus(i).ax= single(0);
      | TOS_AEBLatTargetBus(i).ay= single(0);
      | TOS_AEBLatTargetBus(i).dxVariance= single(0);
      | TOS_AEBLatTargetBus(i).dyVariance= single(0);
      | TOS_AEBLatTargetBus(i).vxVariance= single(0);
      | TOS_AEBLatTargetBus(i).vyVariance= single(0);
      | TOS_AEBLatTargetBus(i).axVariance= single(0);
      | TOS_AEBLatTargetBus(i).ayVariance= single(0);
      | TOS_AEBLatTargetBus(i).ObjectLengthVar= single(0);
      | TOS_AEBLatTargetBus(i).ObjectWidthVar= single(0);
      | TOS_AEBLatTargetBus(i).ObjectYawAngleVar= single(0);
      | TOS_AEBLatTargetBus(i).ObjectTypeProb= single(0);
      | TOS_AEBLatTargetBus(i).ObjectMovingStateProb= single(0);
      | TOS_AEBLatTargetBus(i).ObjectMovingOrientationProb= single(0);
      | TOS_AEBLatTargetBus(i).ObjectExistProb= single(0);
      | TOS_AEBLatTargetBus(i).ObjectIsObstacleProb= single(0);
      | TOS_AEBLatTargetBus(i).ObjectRCS= single(0);
      | TOS_AEBLatTargetBus(i).ObjectMeasurementStatus= single(0);
      | TOS_AEBLatTargetBus(i).ObjectLifeCycle= uint16(0);
      | TOS_AEBLatTargetBus(i).ObjUpdate= false;
      | }
  (junction 47) -> (junction 50) : {i=uint8(1);
      | j=uint8(1);}
  (junction 50) -> (junction 60) [order 1] : [i<=C_TOS_AEBLatTargetSize_Val]
  (junction 48) -> (junction 50) : {i=i+uint8(1);}
  (junction 50) -> (junction 63) [order 2]
  (junction 60) -> (junction 62)
  (junction 62) -> (junction 52) [order 1] : [TOS_AEBLatTargetIndex(i)~=uint8(0)]
  (junction 62) -> (junction 48) [order 2]
  (junction 52) -> (junction 65) : {
      | TargetIndex = TOS_AEBLatTargetIndex(i);
      | TOS_AEBLatTargetBus(j).FusionType=OFM_SignalVerification.Object_Fus_Type(TargetIndex);
      | TOS_AEBLatTargetBus(j).ObjectID=OFM_SignalVerification.Object_ID(TargetIndex);
      | TOS_AEBLatTargetBus(j).ObjectType=AEBLat_TargetObjectType(i);
      | TOS_AEBLatTargetBus(j).ObjectTypeCameraConfirmed=TOS_AddAttributes.PP_CamareConfirmSignalProcessing(TargetIndex);
      | TOS_AEBLatTargetBus(j).ObjectLength=OFM_SignalVerification.Object_Length(TargetIndex);
      | TOS_AEBLatTargetBus(j).ObjectWidth=OFM_SignalVerification.Object_Width(TargetIndex);
      | TOS_AEBLatTargetBus(j).ObjectHight=OFM_SignalVerification.Object_Hight(TargetIndex);
      | TOS_AEBLatTargetBus(j).ObjectYawAngle=OFM_SignalVerification.Object_HeadingAngle(TargetIndex);
      | TOS_AEBLatTargetBus(j).ObjectAzimuthAngle=OFM_SignalVerification.Object_YawAngle(TargetIndex);
      | TOS_AEBLatTargetBus(j).ObjectMovingState=TOS_AddAttributes.PP_MovingState_AEB_SignalProcessing(TargetIndex);
      | TOS_AEBLatTargetBus(j).ObjectMovingOrientation=uint8(3);%Crossing
      | TOS_AEBLatTargetBus(j).dxFisrtDetection=TOS_AddAttributes.PP_ObjFirstDetect_Dx(TargetIndex);
      | TOS_AEBLatTargetBus(j).dyFisrtDetection=TOS_AddAttributes.PP_ObjFirstDetect_Dy(TargetIndex);
      | TOS_AEBLatTargetBus(j).dx=OFM_SignalVerification.Object_DX(TargetIndex);
      | TOS_AEBLatTargetBus(j).dy=OFM_SignalVerification.Object_DY(TargetIndex);
      | TOS_AEBLatTargetBus(j).dz= single(0);
      | TOS_AEBLatTargetBus(j).vx=OFM_SignalVerification.Object_VX(TargetIndex);
      | TOS_AEBLatTargetBus(j).vy=OFM_SignalVerification.Object_VY(TargetIndex);
      | TOS_AEBLatTargetBus(j).ax=OFM_SignalVerification.Object_AX(TargetIndex);
      | TOS_AEBLatTargetBus(j).ay=OFM_SignalVerification.Object_AY(TargetIndex);
      | TOS_AEBLatTargetBus(j).dxVariance=OFM_SignalVerification.Object_Std_DX(TargetIndex);
      | TOS_AEBLatTargetBus(j).dyVariance=OFM_SignalVerification.Object_Std_DY(TargetIndex);
      | TOS_AEBLatTargetBus(j).vxVariance=OFM_SignalVerification.Object_Std_VX(TargetIndex);
      | TOS_AEBLatTargetBus(j).vyVariance=OFM_SignalVerification.Object_Std_VY(TargetIndex);
      | TOS_AEBLatTargetBus(j).axVariance=OFM_SignalVerification.Object_Std_AX(TargetIndex);
      | TOS_AEBLatTargetBus(j).ayVariance=OFM_SignalVerification.Object_Std_AY(TargetIndex);
      | TOS_AEBLatTargetBus(j).ObjectLengthVar=OFM_SignalVerification.Object_Std_Length(TargetIndex);
      | TOS_AEBLatTargetBus(j).ObjectWidthVar=OFM_SignalVerification.Object_Std_Width(TargetIndex);
      | TOS_AEBLatTargetBus(j).ObjectYawAngleVar=OFM_SignalVerification.Object_Std_HeadingAngle(TargetIndex);
      | TOS_AEBLatTargetBus(j).ObjectTypeProb=OFM_SignalVerification.Object_Type_Prob(TargetIndex);
      | TOS_AEBLatTargetBus(j).ObjectMovingStateProb= single(0);
      | TOS_AEBLatTargetBus(j).ObjectMovingOrientationProb= single(0);
      | TOS_AEBLatTargetBus(j).ObjectExistProb=OFM_SignalVerification.Object_ExistProb(TargetIndex);
      | TOS_AEBLatTargetBus(j).ObjectIsObstacleProb=OFM_SignalVerification.Object_ObstacleProb(TargetIndex);
      | TOS_AEBLatTargetBus(j).ObjectRCS= single(0);
      | TOS_AEBLatTargetBus(j).ObjectMeasurementStatus= single(0);
      | TOS_AEBLatTargetBus(j).ObjectLifeCycle=OFM_SignalVerification.Object_Age(TargetIndex);
      | TOS_AEBLatTargetBus(j).ObjUpdate= false;
      | j=j+uint8(1);
      | }
  (junction 65) -> (junction 48)
  data: TOS_AddAttributes input Bus: TOS_AddAttributes_BUS; OFM_SignalVerification input Bus: OFM_OBJ_BUS; AEBLat_TargetObjectType input; TOS_AEBLatTargetIndex input uint8 size=10; TOS_AEBLatTargetBus output Bus: TOS_AEB_LATOBJ_BUS size=10; C_TOS_AEBLatTargetSize_Val parameter; TargetIndex local uint8; i local uint8; j local uint8

== stateflow chart PubIfDecisionTOS_MDL/TOS_20201112/TOS_2012080320/TOS/AEB/TOS_AEBLatCro1105/AEBLat_Object_Condition/AEBLat_TargetCondition/TOS_AEBLat_TargetsDx/Chart ==
  state AEBLatSameTargetIDJudge [function]
    (default) -> (junction 70) : {
        | i = uint8(1);
        | AEBLat_SameTarget = false;
        | }
    (junction 70) -> (junction 81) [order 1] : [i<=C_TOS_AEBLatTargetSize_Val]
    (junction 86) -> (junction 70)
    (junction 70) -> (junction 83) [order 2]
    (junction 81) -> (junction 77)
    (junction 77) -> (junction 78) [order 1] : [AEBLat_Target_ObjectID_K1(i) == Object_ID]
    (junction 77) -> (junction 74) [order 2] : %donothing
    (junction 78) -> (junction 72) : {
        | AEBLat_SameTarget = true;
        | }
    (junction 72) -> (junction 74)
    (junction 74) -> (junction 86) : {i = i+1;}
  (default) -> (junction 1)
  (junction 1) -> (junction 3) [order 1] : [AEBLat_TargetCondition == true]
  (junction 1) -> (junction 97) [order 2] : {
      | TOS_AEBLat_TargetsDx = single(255);
      | }
  (junction 3) -> (junction 88) : {
      | AEBLatSameTargetIDJudge();
      | }
  (junction 88) -> (junction 124) [order 1] : [AEBLat_SameTarget == false]
  (junction 88) -> (junction 94) [order 2] : {
      | TOS_AEBLat_TargetsDx = Object_Dx;
      | }
  (junction 124) -> (junction 114)
  (junction 114) -> (junction 117) [order 1] : [abs(Object_Vy) > P_TOS_CrossingTargetVyvThre_val &&...
      | abs(psiDtOpt) < P_TOS_AEBLatTargetEgoYawRateThre_val]
  (junction 114) -> (junction 118) [order 2] : {
      | TOS_AEBLat_TargetsDx = single(255);
      | }
  (junction 117) -> (junction 112) : {
      | TOS_AEBLat_TargetsDx = Object_Dx;
      | }
  (junction 112) -> (junction 118)
  (junction 118) -> (junction 125)
  (junction 94) -> (junction 97)
  (junction 125) -> (junction 94)
  (junction 97) -> (junction 100)
  data: AEBLat_TargetCondition input boolean; Object_ID input uint8; psiDtOpt input single; AEBLat_Target_ObjectID_K1 input uint8 size=10; Object_Vy input single; TOS_AEBLat_TargetsDx output single size=1; Object_Dx input single; AEBLat_SameTarget local boolean size=1 =false; P_TOS_CrossingTargetVyvThre_val parameter; P_TOS_AEBLatTargetEgoYawRateThre_val parameter; C_TOS_AEBLatTargetSize_Val parameter

== stateflow chart PubIfDecisionTOS_MDL/TOS_20201112/TOS_2012080320/TOS/AEB/TOS_AEBLatCro1105/AEBLat_Object_Condition2/AEBLat_TargetCondition/TOS_AEBLat_TargetsDx/Chart ==
  state AEBLatSameTargetIDJudge [function]
    (default) -> (junction 70) : {
        | i = uint8(1);
        | AEBLat_SameTarget = false;
        | }
    (junction 70) -> (junction 81) [order 1] : [i<=C_TOS_AEBLatTargetSize_Val]
    (junction 86) -> (junction 70)
    (junction 70) -> (junction 83) [order 2]
    (junction 81) -> (junction 77)
    (junction 77) -> (junction 78) [order 1] : [AEBLat_Target_ObjectID_K1(i) == Object_ID]
    (junction 77) -> (junction 74) [order 2] : %donothing
    (junction 78) -> (junction 72) : {
        | AEBLat_SameTarget = true;
        | }
    (junction 72) -> (junction 74)
    (junction 74) -> (junction 86) : {i = i+1;}
  (default) -> (junction 1)
  (junction 1) -> (junction 3) [order 1] : [AEBLat_TargetCondition == true]
  (junction 1) -> (junction 97) [order 2] : {
      | TOS_AEBLat_TargetsDx = single(255);
      | }
  (junction 3) -> (junction 88) : {
      | AEBLatSameTargetIDJudge();
      | }
  (junction 88) -> (junction 124) [order 1] : [AEBLat_SameTarget == false]
  (junction 88) -> (junction 94) [order 2] : {
      | TOS_AEBLat_TargetsDx = Object_Dx;
      | }
  (junction 124) -> (junction 114)
  (junction 114) -> (junction 117) [order 1] : [abs(Object_Vy) > P_TOS_CrossingTargetVyvThre_val &&...
      | abs(psiDtOpt) < P_TOS_AEBLatTargetEgoYawRateThre_val]
  (junction 114) -> (junction 118) [order 2] : {
      | TOS_AEBLat_TargetsDx = single(255);
      | }
  (junction 117) -> (junction 112) : {
      | TOS_AEBLat_TargetsDx = Object_Dx;
      | }
  (junction 112) -> (junction 118)
  (junction 118) -> (junction 125)
  (junction 94) -> (junction 97)
  (junction 125) -> (junction 94)
  (junction 97) -> (junction 100)
  data: AEBLat_TargetCondition input boolean; Object_ID input uint8; psiDtOpt input single; AEBLat_Target_ObjectID_K1 input uint8 size=10; Object_Vy input single; TOS_AEBLat_TargetsDx output single size=1; Object_Dx input single; AEBLat_SameTarget local boolean size=1 =false; P_TOS_CrossingTargetVyvThre_val parameter; P_TOS_AEBLatTargetEgoYawRateThre_val parameter; C_TOS_AEBLatTargetSize_Val parameter

== matlab function PubIfDecisionTOS_MDL/TOS_20201112/TOS_2012080320/TOS/AEB/TOS_AEBLatCro1105/AEBLat_TargetIndex/MATLAB Function ==
  data: Object_Num input; Object_Dx input; ObjDxIndex output
function ObjDxIndex  = fcn(Object_Num, Object_Dx)
ObjNum=int32(80);
ObjDxIndex=uint8(zeros(ObjNum,1));

DxDy=Object_Dx;
MidIndex=int32(1):int32(1):ObjNum;

for i=1:Object_Num
    ObjDxIndex(i)=MidIndex(i);
    t_dis=DxDy(i);
    if i<Object_Num-1
        for j=(i+1):Object_Num
            if DxDy(j)<t_dis
                temp_index=ObjDxIndex(i);
                temp_dis=t_dis;
                
                ObjDxIndex(i)=MidIndex(j);
                DxDy(i)=DxDy(j);
                t_dis=DxDy(j);
                MidIndex(j)=temp_index;
                DxDy(j)=temp_dis;
            end
            
            if DxDy(i) >= single(250)     
                ObjDxIndex(i)=uint8(0); 
            end           
   
        end
    else
        if i~=Object_Num
            if DxDy(Object_Num)<t_dis
                temp_index=ObjDxIndex(i);
                temp_dis=t_dis;
                ObjDxIndex(i)=MidIndex(Object_Num);
                DxDy(i)=DxDy(Object_Num);
                MidIndex(Object_Num)=temp_index;
                DxDy(Object_Num)=temp_dis;
            else
                MidIndex(Object_Num)=MidIndex(Object_Num);
                DxDy(Object_Num)=DxDy(Object_Num);
            end
            
            if DxDy(i) >= single(250)     
                ObjDxIndex(i)=uint8(0); 
            end       
            
        end
    end

end

== stateflow chart PubIfDecisionTOS_MDL/TOS_20201112/TOS_2012080320/TOS/AEB/TOS_AEBLatCro_20201208/AEBLatTrgInfor/AEBLatTargetObjectType/AEBLatTargetObjectType/TOS_AEBLat_TargetObjectType ==
  state AEBLatSameTargetType [function]
    (default) -> (junction 39) : {
        | i = uint8(1);
        | AEBLat_TargetObjectType = OFM_OBJ_TYPE_E.INVALID;
        | }
    (junction 39) -> (junction 40) [order 1] : [i<=C_TOS_AEBLatTargetSize_Val]
    (junction 45) -> (junction 39)
    (junction 39) -> (junction 46) [order 2]
    (junction 40) -> (junction 41)
    (junction 41) -> (junction 42) [order 1] : [AEBLat_Target_ObjectID_K1(i) == Object_ID]
    (junction 41) -> (junction 43) [order 2] : %donothing
    (junction 42) -> (junction 44) : {
        | AEBLat_TargetObjectType = AEBLat_Target_ObjectType_K1(i);
        | i = C_TOS_AEBLatTargetSize_Val+uint8(1);
        | }
    (junction 44) -> (junction 43)
    (junction 43) -> (junction 45) : {i = i+uint8(1);}
  (default) -> (junction 1)
  (junction 1) -> (junction 5) [order 1] : [ObjectType == OFM_OBJ_TYPE_E.PEDESTRIAN||...
      | ObjectType == OFM_OBJ_TYPE_E.BICYCLE||...
      | ObjectType == OFM_OBJ_TYPE_E.MOTORBIKE]
  (junction 1) -> (junction 27) [order 2] : {
      | AEBLatSameTargetType();
      | }
  (junction 5) -> (junction 26) : {
      | AEBLat_TargetObjectType = ObjectType;
      | }
  (junction 26) -> (junction 27)
  (junction 27) -> (junction 30)
  data: Object_ID input uint8; ObjectType input; AEBLat_Target_ObjectType_K1 input Enum: OFM_OBJ_TYPE_E; AEBLat_Target_ObjectID_K1 input uint8; AEBLat_TargetObjectType output Enum: OFM_OBJ_TYPE_E; C_TOS_AEBLatTargetSize_Val parameter
